simulink library "INT_DevLib_ActrPrt"  (R2016b)
settings: Solver=VariableStepAuto  StartTime=0.0  StopTime=10.0  RelTol=1e-3
settings Model: Creator=Administrator  LastModifiedBy=Administrator

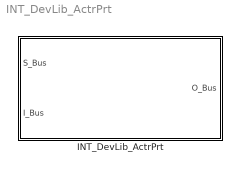
== system INT_DevLib_ActrPrt ==
  INT_DevLib_ActrPrt : Subsystem

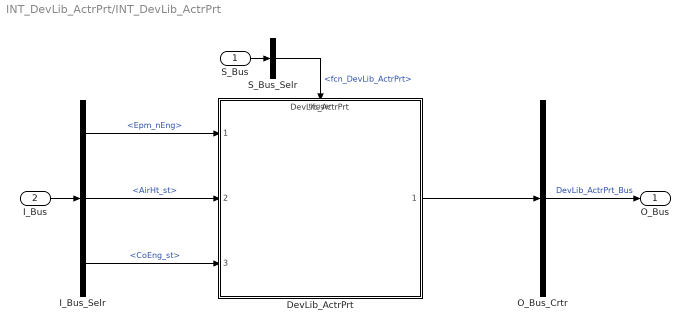
== system INT_DevLib_ActrPrt/INT_DevLib_ActrPrt ==
  S_Bus : Inport
  I_Bus : Inport  Port=2
  DevLib_ActrPrt : ModelReference  ModelNameDialog=DevLib_ActrPrt  SimulationMode=Normal  ModelReferenceVersion=1.7  TriggerPortName=function  TriggerPortTriggerType=function-call  TriggerPortStatesWhenEnabling=held
  I_Bus_Selr : BusSelector  OutputSignals=Epm_nEng,AirHt_st,CoEng_st
  O_Bus_Crtr : BusCreator  Inputs=1
  S_Bus_Selr : BusSelector  OutputSignals=fcn_DevLib_ActrPrt
  O_Bus : Outport
  wires:
  S_Bus_Selr/1 -> DevLib_ActrPrt/Trigger  "<fcn_DevLib_ActrPrt>"
  S_Bus/1 -> S_Bus_Selr/1
  I_Bus/1 -> I_Bus_Selr/1
  I_Bus_Selr/1 -> DevLib_ActrPrt/1  "<Epm_nEng>"
  I_Bus_Selr/2 -> DevLib_ActrPrt/2  "<AirHt_st>"
  I_Bus_Selr/3 -> DevLib_ActrPrt/3  "<CoEng_st>"
  O_Bus_Crtr/1 -> O_Bus/1  "DevLib_ActrPrt_Bus"
  DevLib_ActrPrt/1 -> O_Bus_Crtr/1
